simulink model "ANC_try1"  (R2016b)
settings: Solver=ode45  StartTime=0.0  StopTime=10  RelTol=1e-3  EnableMultiTasking=on
libraries: dspvision x1, dspadpt3 x1, dspsrcs4 x1, dspobslib x1
settings Model: Creator=Aalim  LastModifiedBy=pangaq
settings DataIOCC: LimitDataPoints=on  SaveFormat=Array
settings OptimizationCC: ExpressionDepthLimit=2147483647  LifeSpan=inf
settings DebuggingCC: UnderspecifiedInitializationDetection=Classic  MergeDetectMultiDrivingBlocksExec=none  SolverPrmCheckMsg=warning  StateNameClashWarn=warning  SFUnexpectedBacktrackingDiag=warning  SFNoUnconditionalDefaultTransitionDiag=warning  SFExecutionAtInitializationDiag=none
settings HardwareCC: ProdBitPerPointer=32  ProdBitPerSizeT=32  ProdBitPerPtrDiffT=32  ProdLargestAtomicFloat=None  ProdIntDivRoundTo=Undefined  ProdEndianess=Unspecified  ProdWordSize=32  ProdHWDeviceType=32-bit Generic
settings ModelReferenceCC: PropagateSignalLabelsOutOfModel=off
settings GRTTargetCC: TargetLangStandard=C89/C90 (ANSI)  GeneratePreprocessorConditionals=Disable all
settings ConfigComp: CovMetricSettings=dw  CovHtmlReporting=on  CovSaveCumulativeToWorkspaceVar=on  CovSaveSingleToWorkspaceVar=on  CovExternalEMLEnable=off

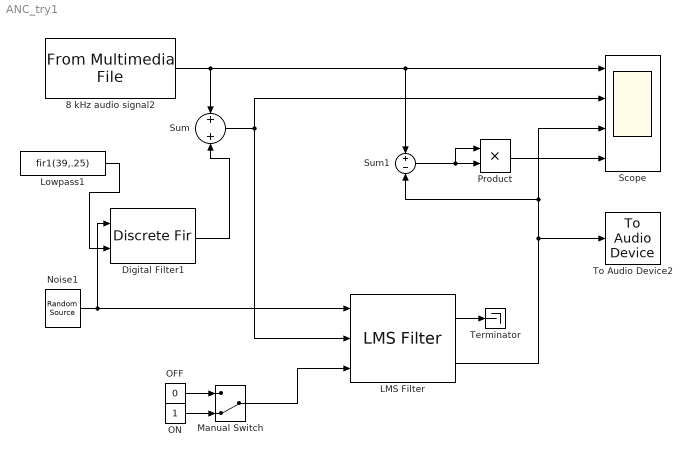
== system ANC_try1 ==
  8 kHz audio signal2 : dspvision/From Multimedia File  inputFilename=E:\belltone.wav  loop=on  numPlays=inf  outputStreams=Audio only  videoDataType=single  audioDataType=single  inheritSampleTime=off  userDefinedSampleTime=1/250  noAudioOutput=off  isIntensityVideo=off  fourcc=RGB  colorVideoFormat=Separate color signals  outputEOF=off  dataOrg=Column-major  audioFrameSize=32  computeAudioFrameSize=off  outSamplingMode=Sample based
  Digital Filter1 : DiscreteFir  CoefSource=Input port  Coefficients=[1 2]  InputProcessing=Columns as channels (frame based)  AccumDataTypeStr=Inherit: Same as product output  OutDataTypeStr=Inherit: Same as input
      settings: InputPortMap=u0,u1
  LMS Filter : dspadpt3/LMS Filter  Algo=LMS  L=32  stepflag=Dialog  mu=0.0008  leakage=1.0  ic=0  Adapt=on  resetflag=None  weights=off  secondCoeffMode=User-defined  secondCoeffWordLength=2  secondCoeffFracLength=15  accum2Mode=User-defined  accum2FracLength=20  prodOutput2Mode=User-defined  prodOutput2FracLength=20  prodOutput3Mode=User-defined  prodOutput3FracLength=20  prodOutput4Mode=User-defined  prodOutput4FracLength=20  quotientMode=User-defined  quotientFracLength=20  roundingMode=Floor  overflowMode=off  addnparflag=off
  Lowpass1 : Constant  Value=fir1(39,.25)  OutDataTypeStr=Inherit: Inherit via back propagation
  Manual Switch : ManualSwitch  CurrentSetting=0
  Noise1 : dspsrcs4/Random Source  SrcType=Gaussian  NormMethod=Sum of uniform values  CltLength=5  MinVal=-1  MaxVal=1  MeanVal=0  VarVal=1  RepMode=Specify seed  rawSeed=[23341]  IsInherit=off  SampMode=Discrete  SampTime=1/8000  SampFrame=32  DataType=Single  OutComplex=Real  OutputFrames=off
  OFF : Constant  Value=0
  ON : Constant
  Product : Product  RndMeth=Zero
  Scope : Scope  NumInputPorts=4
  Sum : Sum  Inputs=+|+
  Sum1 : Sum  Inputs=+|-
  Terminator : Terminator
  To Audio Device2 : dspobslib/To Audio Device  deviceName=Primary Sound Driver  inheritSampleRate=on  sampleRate=44100  deviceDatatype=Determine from input data type  autoBufferSize=on  bufferSize=4096  queueDuration=1.0  defaultOutputChannelMapping=on  outputChannelMapping=1:2  outputNumUnderrunSamples=off
  wires:
  8 kHz audio signal2/1 -> Scope/1, Sum1/1, Sum/1
  Sum/1 -> LMS Filter/2, Scope/2
  Noise1/1 -> Digital Filter1/1, LMS Filter/1
  LMS Filter/1 -> Terminator/1
  LMS Filter/2 -> To Audio Device2/1, Scope/3, Sum1/2
  Sum1/1 -> Product/2, Product/1
  Digital Filter1/1 -> Sum/2
  Product/1 -> Scope/4
  OFF/1 -> Manual Switch/1
  ON/1 -> Manual Switch/2
  Manual Switch/1 -> LMS Filter/3
  Lowpass1/1 -> Digital Filter1/2
